simulink model "module_2018"  (R2018b)
settings: Solver=FixedStepAuto  StartTime=0.0  StopTime=10.0  RelTol=1e-3
settings Model: Creator=lenovo  LastModifiedBy=lenovo
settings DataIOCC: SaveOutput=off  ReturnWorkspaceOutputs=on
settings DebuggingCC: UnderSpecifiedDimensionMsg=warning

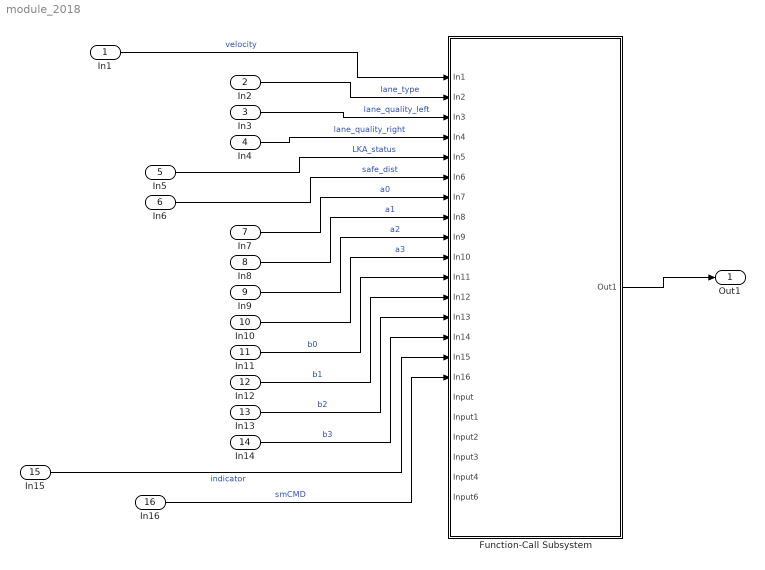
== system module_2018 ==
  In1 : Inport
  In2 : Inport  Port=2
  In3 : Inport  Port=3
  In4 : Inport  Port=4
  In5 : Inport  Port=5
  In6 : Inport  Port=6
  In7 : Inport  Port=7
  In8 : Inport  Port=8
  In9 : Inport  Port=9
  In10 : Inport  Port=10
  In11 : Inport  Port=11
  In12 : Inport  Port=12
  In13 : Inport  Port=13
  In14 : Inport  Port=14
  In15 : Inport  Port=15
  In16 : Inport  Port=16
  Function-Call Subsystem : Subsystem  TreatAsAtomicUnit=on
  Out1 : Outport
  wires:
  Function-Call Subsystem/1(Out1) -> Out1/1
  In2/1 -> Function-Call Subsystem/2(In2)  "lane_type"
  In8/1 -> Function-Call Subsystem/8(In8)  "a1"
  In7/1 -> Function-Call Subsystem/7(In7)  "a0"
  In1/1 -> Function-Call Subsystem/1(In1)  "velocity"
  In3/1 -> Function-Call Subsystem/3(In3)  "lane_quality_left"
  In5/1 -> Function-Call Subsystem/5(In5)  "LKA_status"
  In4/1 -> Function-Call Subsystem/4(In4)  "lane_quality_right"
  In12/1 -> Function-Call Subsystem/12(In12)  "b1"
  In6/1 -> Function-Call Subsystem/6(In6)  "safe_dist"
  In10/1 -> Function-Call Subsystem/10(In10)  "a3"
  In11/1 -> Function-Call Subsystem/11(In11)  "b0"
  In9/1 -> Function-Call Subsystem/9(In9)  "a2"
  In14/1 -> Function-Call Subsystem/14(In14)  "b3"
  In15/1 -> Function-Call Subsystem/15(In15)  "indicator"
  In16/1 -> Function-Call Subsystem/16(In16)  "smCMD"
  In13/1 -> Function-Call Subsystem/13(In13)  "b2"

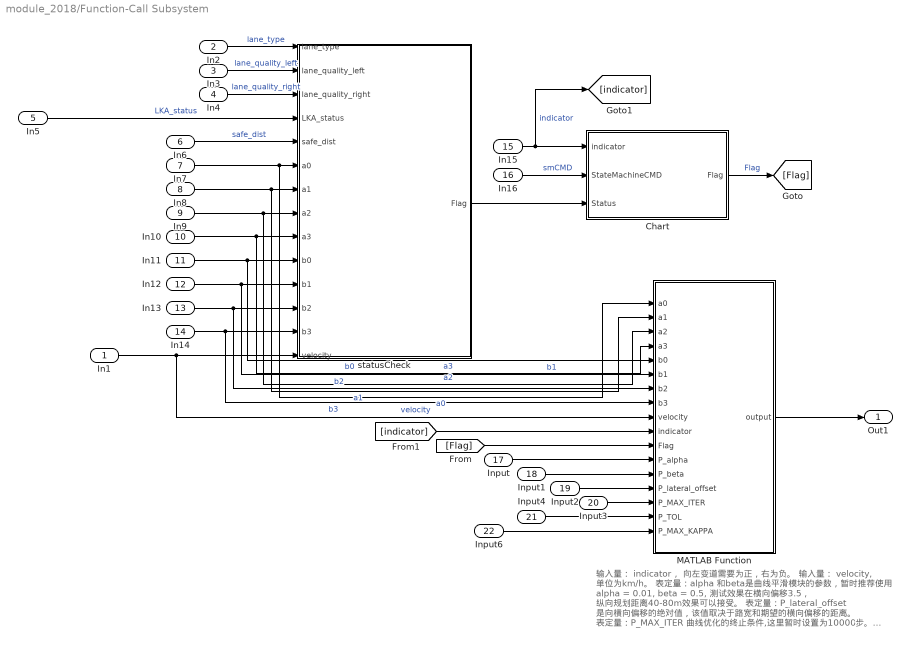
== system module_2018/Function-Call Subsystem ==
  note: 输入量： indicator， 向左变道需要为正，右为负。
      | 输入量： velocity, 单位为km/h。
      |
      | 表定量：alpha 和beta是曲线平滑模块的参数，暂时推荐使用 alpha = 0.01, beta = 0.5, 测试效果在横向偏移3.5，
      |  纵向规划距离40-80m效果可以接受。
      | 表定量：P_lateral_offset 是向横向偏移的绝对值，该值取决于路宽和期望的横向偏移的距离。
      | 表定量：P_MAX_ITER 曲线优化的终止条件,这里暂时设置为10000步。
      | 表定量：P_TOL 优化后的曲线与原曲线之间可以接受的最大偏移量，这里推荐使用0.7m
      | 表定量：P_MAX_KAPPA 曲线的优化目标，希望将曲线的曲率下降到某个值以下，这里推荐是用0.002,也就是曲率半径500m.
  In1 : Inport
  In2 : Inport  Port=2
  In3 : Inport  Port=3
  In4 : Inport  Port=4
  In5 : Inport  Port=5
  In6 : Inport  Port=6
  In7 : Inport  Port=7
  In8 : Inport  Port=8
  In9 : Inport  Port=9
  In10 : Inport  Port=10
  In11 : Inport  Port=11
  In12 : Inport  Port=12
  In13 : Inport  Port=13
  In14 : Inport  Port=14
  In15 : Inport  Port=15
  In16 : Inport  Port=16
  Input : Inport  Port=17
  Input1 : Inport  Port=18
  Input2 : Inport  Port=19
  Input3 : Inport  Port=20
  Input4 : Inport  Port=21
  Input6 : Inport  Port=22
  Chart : Stateflow chart  TreatAsAtomicUnit=on
  MATLAB Function : MATLAB Function  TreatAsAtomicUnit=on
  "statusCheck " : MATLAB Function  TreatAsAtomicUnit=on
  Out1 : Outport
  wires:
  In1/1 -> "statusCheck "/14(velocity), MATLAB Function/9(velocity)  "velocity"
  In2/1 -> "statusCheck "/1(lane_type)  "lane_type"
  In3/1 -> "statusCheck "/2(lane_quality_left)  "lane_quality_left"
  In4/1 -> "statusCheck "/3(lane_quality_right)  "lane_quality_right"
  In6/1 -> "statusCheck "/5(safe_dist)  "safe_dist"
  In7/1 -> MATLAB Function/1(a0), "statusCheck "/6(a0)  "a0"
  In5/1 -> "statusCheck "/4(LKA_status)  "LKA_status"
  In8/1 -> MATLAB Function/2(a1), "statusCheck "/7(a1)  "a1"
  In10/1 -> MATLAB Function/4(a3), "statusCheck "/9(a3)  "a3"
  In11/1 -> MATLAB Function/5(b0), "statusCheck "/10(b0)  "b0"
  In9/1 -> MATLAB Function/3(a2), "statusCheck "/8(a2)  "a2"
  In12/1 -> MATLAB Function/6(b1), "statusCheck "/11(b1)  "b1"
  In14/1 -> MATLAB Function/8(b3), "statusCheck "/13(b3)  "b3"
  In13/1 -> MATLAB Function/7(b2), "statusCheck "/12(b2)  "b2"
  MATLAB Function/1(output) -> Out1/1
  "statusCheck "/1(Flag) -> Chart/3(Status)
  In15/1 -> [indicator], Chart/1(indicator)  "indicator"
  In16/1 -> Chart/2(StateMachineCMD)  "smCMD"
  Chart/1(Flag) -> [Flag]  "Flag"
  [Flag] -> MATLAB Function/11(Flag)
  [indicator] -> MATLAB Function/10(indicator)
  Input/1 -> MATLAB Function/12(P_alpha)
  Input1/1 -> MATLAB Function/13(P_beta)
  Input2/1 -> MATLAB Function/14(P_lateral_offset)
  Input3/1 -> MATLAB Function/15(P_MAX_ITER)
  Input4/1 -> MATLAB Function/16(P_TOL)
  Input6/1 -> MATLAB Function/17(P_MAX_KAPPA)

== matlab function module_2018/Function-Call Subsystem/statusCheck  ==
  data: lane_type input; Flag output; lane_quality_left input; lane_quality_right input; LKA_status input; safe_dist input; a0 input; a1 input; a2 input; a3 input; b0 input; b1 input; b2 input; b3 input; velocity input
function Flag = functionisOK(lane_type, lane_quality_left, lane_quality_right, ...
    LKA_status,safe_dist,a0,a1,a2,a3, b0,b1,b2,b3,velocity)
%% this function provides a status check method, only when the status check Flag = 1, 
% can the lane change method is activated. 
% we consider the follow 5 terms to demtermine whether the method can be
% activated;
% 1. lane type, we can only change lane when the type is dashed line
%2, lane quality, we only allow lane change when left and right lane
%quality is ok;
% 3. LKA status is the pre-requisite that lane changing method can be
% activated;
% 4. safe_dist comes from ACC module, we only allow lane change when the
% front vehicle safety distance is big enough to ensure safety space for
% lane changing;
% 5. kappa is the both the left and right lane curvature, which means only
% when the kappa is big enough, very close to straight line, can we
% activate lane changing method;
    LEN = calculateLEN(velocity)
    lane_type_flag = 0;
    lane_quality_flag = 0;
    LKA_status_flag = 0;
    safe_dist_flag = 0;
    
    
    if lane_type == 1
        lane_type_flag = 1;
    end
    
    if (lane_quality_left >=3) && (lane_quality_right >=3)
        lane_quality_flag = 1; 
    end
    
    if LKA_status == 1
        LKA_status_flag = 1;
    end
    
    if safe_dist > 0.2 * LEN
        safe_dist_flag = 1;
    end
    
    
    y_d=  [0];
    y_dd = [0];
    kappa = [0];
    for i = 1:round(LEN)
        y_d = [y_d, a1 + 2*a2*i + 3*a3*i^2];
        y_dd = [y_dd, 2*a2 + 6*a3*i];
    end
    
    for i = 1:length(y_d)
        kappa(i)=  y_dd(i) / ((1 + (y_d(i))^2)^(1.5));
    end
    plot(1:length(y_d), kappa)
    
    for i = 1: length(kappa)
        if abs(kappa(i))> 1/250
            kappa_flag = 0;
            break;
        else
            kappa_flag = 1;
        end
    end
    
   if((lane_type_flag == 1) && (lane_quality_flag == 1) && (LKA_status_flag == 1)...
       && (kappa_flag == 1) && (safe_dist_flag == 1))
       Flag = 1;
   else
       Flag = 0;
   end
   
end

function LEN = calculateLEN(velocity)
    LEN = velocity;
end

== matlab function module_2018/Function-Call Subsystem/MATLAB Function ==
  data: a0 input; output output size=1000; a1 input; a2 input; a3 input; b0 input; b1 input; b2 input; b3 input; velocity input; indicator input; Flag input; P_alpha input; P_beta input; P_lateral_offset input; P_MAX_ITER input; P_TOL input; P_MAX_KAPPA input
function output = LineGeneration(a0,a1,a2,a3, b0,b1,b2,b3,velocity,indicator,Flag,P_alpha,P_beta,P_lateral_offset,...
    P_MAX_ITER,P_TOL, P_MAX_KAPPA )
%% the main function, which is used to generate changing lane curve dynamically    
    if Flag ~= 2
        output = [];
        return;
    end
    
    LEN = calculateLEN(velocity);
    reference_1 = reference_line_generator(a0,a1,a2,a3, b0,b1,b2,b3,LEN);
    S = 0;
    D0 = 0.5 * (a0 + b0);
    Ti = LEN;
    Di = abs(P_lateral_offset) * indicator;% indicator signal should be positive when turning left, and vice versa.
    [ref_bezier] = ref_bezier_generation(reference_1, D0,Ti,Di);
    trajs_new_origin = reference_generation(reference_1, ref_bezier);
    trajs_new = PathSmoothing(trajs_new_origin, P_alpha, P_beta,P_MAX_ITER,P_TOL, P_MAX_KAPPA);
    delta_heading_rad = calculat_delta_heading(reference_1, trajs_new);
    delta_heading_deg = rad_to_deg(delta_heading_rad);
    kappa = calculate_kappa(trajs_new);
    output = [ref_bezier,delta_heading_rad,kappa];
end

function LEN = calculateLEN(velocity)
    LEN = velocity;
    LEN = round(LEN);
    
    if LEN == 0
        fprintf('LEN calculation error. \r')
    end
end

function [ref_bezier] = ref_bezier_generation(reference_1, D0, Ti, Di)
%% this function generate bezier curve information 
% input: the centerline reference_1, bezier curve control points
% output: the matrix is in dimension of n by 2, with its first col
% longitudinal integration length, second col lateral offset with respect
% to center line.
% notice: shifting to left is positive, and vice versa. 
S = 0;
    ref_bezier = [[],[]];
    index =1;
    while S < Ti
        p = Bezierfrenet_5(D0, Ti, Di,S);
        ref_bezier =[ref_bezier; p];
        S = S + sqrt((reference_1(index+1,1)-reference_1(index,1))^2 + ...
            (reference_1(index+1,2)-reference_1(index,2))^2);
        index = index + 1;
    end
end

function [delta_heading] = calculat_delta_heading(center_line, traj_new)
    LEN = min(length(center_line), length(traj_new));
    delta_heading = [0];
    for i = 1: LEN-1
        x1 = center_line(i+1,1) - center_line(i,1);
        y1 = center_line(i+1,2) - center_line(i,2);
        x2 = traj_new(i+1,1) - traj_new(i,1);
        y2 = traj_new(i+1,2) - traj_new(i,2);
        delta_theta =  (x1 * x2 + y1 * y2) / (sqrt(x1^2 + y1^2) * sqrt(x2^2 + y2^2));
        delta_heading =  [delta_heading; acos(delta_theta)];
    end
end

function [reference] = reference_line_generator(a0,a1,a2,a3, b0,b1,b2,b3, LEN)
%% in this function, we use the left and right lane polynomials to generate
% a reference center line
% input: left lane polynomials, right lane polynomials, LEN(length of reference)
% output: reference center line polynomials
reference = [[],[]];
if LEN == 0
    fprintf('LEN = 0, reference cannot be generated. \r')
    return;
end

for i = 0:0.2:LEN
    y = 0.5 * ( (a0 + a1 * i + a2 * i^2 + a3 * i^3) + (b0 + b1 * i + b2 * i^2 + b3 * i^3));
    reference =  [reference; [i,y]];
end
end

function y = f_a(a0, a1, a2, a3, x)
%% calculate polynomial y values
    y = a0 + a1 * x + a2 * x^2 + a3 * x^3;
end

function y = f_b(b0, b1, b2, b3, x)
%% calculate polynomial y values
    y = b0 + b1 * x + b2 * x^2 + b3 * x^3;
end

function y = deg_to_rad(x)
%% deg to rad unit switch
    y = x * pi / 180;
end

function y = rad_to_deg(x)
%% rad to degree unit switch
    y = x * 180 / pi;
end

function [reference] = reference_line_generator_frenet(a0,a1,a2,a3, b0,b1,b2,b3, LEN)
%% this function generates center line in discrete form
% input: the left lane and right lane polynomials parameters, and
% longitudinal LEN(how long we want to generate such a curve)
% output: using frenet method to generate the ceterline position in x and
% y

if LEN == 0
    fprintf('LEN = 0, reference cannot be generated. \r');
    return;
end

S = 0;
iter = 0;
x_a = 0;
x_b = 0;

delta_x = 0.02;
RESOLUTION = 0.2;
y_a_pre = f_a(a0,a1,a2,a3, x_a);
y_b_pre = f_b(b0,b1,b2,b3, x_b);
reference = [x_a, 0.5*(y_a_pre + y_b_pre)];
while S < LEN

    s_a = 0;
    s_b = 0;
    while s_a < RESOLUTION
        x_a = x_a + delta_x;
        y_a = f_a(a0,a1,a2,a3, x_a);
        s_a = s_a + sqrt( delta_x^2 + (y_a - y_a_pre)^2);
        y_a_pre = y_a;
    end
    
    while s_b < RESOLUTION 
        x_b = x_b + delta_x;
        y_b = f_b(b0,b1,b2,b3, x_b);
        s_b = s_b + sqrt( delta_x^2 + (y_b - y_b_pre)^2);
        y_b_pre = y_b;
    end
    
    S = S + RESOLUTION;
    reference = [reference; [0.5*(x_a + x_b), 0.5*(y_a + y_b) ]];
    
    iter = iter + 1;
    if iter >= 5000
        print("while loop too long, missing error! \r")
        break;
    end
    
end
end

function [p] = Bezierfrenet_5(D0, Ti, Di,t)
%% this function provides the bezier curve information. 
% when given control points information, it can generate y values based on
% given x values.
    p0 = [ 0, D0];
    p1 = [0.25 * Ti, D0];
    p2= [0.5 *Ti, D0];
    p3 =[ 0.5 * Ti, Di];
    p4 =[ 0.75 * Ti, Di];
    p5 = [Ti, Di];
  %generate a fifth order bezier curve

    p= (1-(t)/Ti)^5*p0 + 5*(1-(t)/Ti)^4*((t)/Ti)*p1 + 10*(1-(t)/Ti)^3*((t)/Ti)^2*p2 +...
     10*(1-(t)/Ti)^2*((t)/Ti)^3*p3 +5*(1-(t)/Ti)*((t)/Ti)^4*p4 + ((t)/Ti)^5*p5;

end
 
function [trajs_new] = reference_generation(trajs_local, p_store)
%% this function provides method of generating changing lane discrete positions.    
% inputs: here the trajs_local is a vector<vector<double>>,with its dimension
%n by 2, the p_store store the information Bezier curve generaion
%function creates, which are longitudinal 's' and 'lateral offset', which
%is also in dimension of n by 2. 
%output: with the two inputs info, we are able to generate under vehicle
%coordinate the changing lane positions by doing position shift, based on
%the original trajs_local, in frenet direction with offset info provided by
%p_store.
if (isempty(trajs_local)) || (length(trajs_local) == 0)
    fprintf('reference trajs is not well generated! \r');
    trajs_new= [];
    return;
end

if isempty(p_store) || (length(p_store) == 0)
    fprintf('offset Bezier curve is not well generated! \r');
    trajs_new= [];
    return;
end

    trajs_new = [[ ],[ ]];
    for i = 1: min(length(p_store), length(trajs_local))
%         if (i + current_index) > length(waypoint)
%             break;
%         end
        d = p_store(i,2);
        if trajs_local(i,1) == 0
            theta = 0;
        else
            theta = atan(trajs_local(i,2) / trajs_local(i,1));
        end
        
        if (theta>-pi/2 && theta <=0)
            x = trajs_local(i,1) - d * sin(theta);
            y = trajs_local(i,2) + d * cos(theta);
            trajs_new = [trajs_new ; [x,y]];
        elseif (theta>0 && theta < pi/2)
            x = trajs_local(i,1) - d * sin(theta);
            y = trajs_local(i,2) + d * cos(theta);
            trajs_new = [trajs_new ; [x,y]];    
        else
           fprintf("it seems that the reference line is unacceptable!");
        end
    end
end

function optPath = PathSmoothing(path, alpha, beta,P_MAX_ITER,P_TOL, P_MAX_KAPPA)
    optPath=path;%
    iter = 0;
    COND = 1;
    while COND == 1 
%         change=0;
        for ip=2:(length(path(:,1))-1) 
          optPath(ip,:)=optPath(ip,:)-alpha*(optPath(ip,:)-path(ip,:));
            term_dx_1 = 2*optPath(ip,:)-optPath(ip-1,:)-optPath(ip+1,:);
%             term_dx_2 = optPath(ip-2,:) - 4*optPath(ip-1,:) + 6 * optPath(ip,:)...
%                 -4 * optPath(ip+1,:) - optPath(ip+2,:);
            optPath(ip,:) = optPath(ip,:)-beta * term_dx_1;
%           change=change+norm(optPath(ip,:)-prePath);
        end
        kappa = calculate_kappa(optPath);
        
        iter = iter + 1
        
        change = zeros(1,length(optPath));
        for i = 1:length(optPath)
            change(i) = norm(optPath(i,:)-path(i,:));
            if max(abs(change)) >= P_TOL % 0.7
                COND = 2
                 [value, loc] = max(abs(change))
                break;
            end
        end
        
        if iter > P_MAX_ITER % 10000
            COND = 3;
        end
        
        sum = 0;
        for i = 1: length(kappa)    
            if abs(kappa(i)) > P_MAX_KAPPA %0.002
               sum = sum + 1; 
            end
        end
        
        if sum == 0
            COND = 4
        end
                   
    end
end


function [kappa] = calculate_kappa(trajs_new)

%% this function provide the method of generating a sequence of curvature(kappa) 
% input: a sequence of discrete points with position x and y.
% output: a sequence of kappa on each point.
% notice: vehicle turning right has negative curvature, and vice versa.

if (isempty(trajs_new)) || (length(trajs_new) == 0)
    fprintf('changing lane trajs is not well generated! \r');
    kappa = zeros(length(trajs_new),1);
    return;
end

    pd = zeros(length(trajs_new),1);
    pdd = zeros(length(trajs_new),1);
    kappa = zeros(length(trajs_new),1);
    
    % calculate the first derivatives
    
    for i = 1:length(trajs_new)-1
        
        if (trajs_new(i+1,1)-trajs_new(i,1)) == 0
            denominator_pd = 0.001;
        else
            denominator_pd = trajs_new(i+1,1)-trajs_new(i,1);
        end
        
        pd(i) = (trajs_new(i+1,2)-trajs_new(i,2))/denominator_pd;   
    end
    pd(length(trajs_new)) = pd(length(trajs_new)-1);
    % calculate the second derivatives
    pdd(1) = 0;
    for i =2: length(trajs_new)-1
        
        if (0.5*(-trajs_new(i-1,1)+trajs_new(i+1,1)))^2 == 0
            denominator_pdd = 0.001;
        else
            denominator_pdd = 0.5*(-trajs_new(i-1,1)+trajs_new(i+1,1))^2;
        end
        
        pdd(i) = (trajs_new(i+1,2)-2*trajs_new(i,2) +...
            trajs_new(i-1,2))/denominator_pdd;
    end
    pdd(length(trajs_new)) = pdd(length(trajs_new)-1);
    
    for i  = 1:length(trajs_new)
        kappa(i) = (pdd(i))/((1+pd(i)^2)^(1.5));
    end
end

function [location] = update_trajs(velocity,trajs_new,delta_t)
%% this function dynamically update trajs_new for LKA system
S = velocity * delta_t;
    s = 0;
    for i = 1: length(trajs_new)
        s = s + sqrt((trajs_new(i+1,1) - trajs_new(i,1))^2 + ...
            (trajs_new(i+1,2) - trajs_new(i,2))^2);
        if s>= S
            break;
        end
    end
end

== stateflow chart module_2018/Function-Call Subsystem/Chart ==
  state Standby
    du:
    Flag = 1;
  state OFF
    entry:
    Flag = 0;
  state Run
    du:
    Flag = 2;
  Standby -> OFF [order 2] : [indicator == 0]
  OFF -> Standby : [Status == 1]
  (default) -> OFF
  Standby -> Run [order 1] : [StateMachineCMD == 1 && indicator == 1]
  Run -> Standby : [StateMachineCMD == 0 || indicator == 0]
  data: Flag output; indicator input; StateMachineCMD input; Status input
